simulink model "Aero_Workspace"  (R2021a)
settings: Solver=ode1be  StartTime=0.0  StopTime=inf  FixedStep=0.001  RelTol=1e-3  EnableMultiTasking=on
PreLoadFcn:
  | Aero_Workspace_Setup
model workspace (MAT data in the model file):
  Dg = 0.0071
  Dt = 0.158
  Jp = 0.022
  Mb = 1.3
  g = 9.81
values from neighbouring files (symbols this model uses):
  Kpp = 0.6*0.0154    (= 0.00924)    [Aero_Workspace_Parameters.m]
  Kpy = 2*0.00329    (= 0.00658)    [Aero_Workspace_Parameters.m]
  Kyp = -2.5*0.00167    (= -0.004175)    [Aero_Workspace_Parameters.m]
  Kyy = 0.0129    [Aero_Workspace_Parameters.m]
  Pitch_deg_range = 62    [Aero_Workspace_Setup.m]
undefined symbols (not defined in the file or in its folder): _AICAD8418WBRMZ_Default_sldprt, _AICBCR421UW67_Default_sldprt, _C0402100n25V_Default_sldprt, _C040210n25V_Default_sldprt, _C040212p50VC0G_Default_sldprt, _C06031u35V_Default_sldprt, _C06032u216V_Default_sldprt, _C100U50VEEEFC1H101P_Default_sldprt, _C12064u750V_01_sldprt, _C121010U50V_Default_sldprt, _COMMCYUSB2014BZXC_Default_sldprt, _COMMON_01_sldprt, _COMMON_Default_sldprt, _CONNFUSBBSMT_01_sldprt, _CONNMDF3A12P2DSA_Default_sldprt, _CONNMDF3A4P2DSA_Default_sldprt, _CONNMDF3A6P2DS_Default_sldprt, _CONNMDF3A9P2DS_Default_sldprt, _CONNMODULAR8P8CTOP_Default_sldprt, _CP6100U50VC0G_Default_sldprt, _CPLD5M80ZE64C5_Default_sldprt, _DB560C13F_01_sldprt, _Default_sldprt, _DSMBJ5361BTP_Default_sldprt, _EEPROMAT24CM01_Default_sldprt, _FBBLM21PG221SN1D_01_sldprt, _FBMPZ2012S601A_01_sldprt, _LED3mmRedGreenRA_Default_sldprt, _LEDLTRBGFSFRedGreenBlue_Default_sldprt, _LOGICNCP361SNT1G_Default_sldprt, _LOGICNOTSN74LVC3G14DCU_Default_sldprt, _OPL6206QTR_Default_sldprt, _OSC40000MHZ_Default_sldprt, _R0402100K_Default_sldprt, _R040210K0_Default_sldprt, _R04021K00_Default_sldprt, _R0402200R_Default_sldprt, _R040222R0_Default_sldprt, _R04026K04_Default_sldprt, _R0402DNP_Default_sldprt, _RA40R0_Default_sldprt, _RA41K005, _TP16258543_01_sldprt, _TVSUNI28V_Default_sldprt, _TVSUNI53V_Default_sldprt, _VREGAP733333SAG7_Default_sldprt, _VREGLTM8022EVPBF_Default_sldprt, _VREGPAM3112DAB120_Default_sldprt, _VREGTPS79318DBVR_01_sldprt, _XTAL192MHZNX2520SA_Default_sldprt, BGA121, CAP, CEEEFC1H101P, CONNFUSBBSMT, CONNMDF3A12P2DSA, CONNMDF3A4P2DSA, CONNMDF3A6P2DS, CONNMDF3A9P2DS, CONNModular8P8C, DDO214AA ... (+30)
libraries: sm_lib x1565, fl_lib x43, nesl_utility x22, quarc_library x12, simulink x2, ee_lib x2
(part 1 of 23)
settings Model: SimulationMode=external  ExtModeTrigDuration=10000  OrderedModelArguments=off  Creator=mbohra  LastModifiedBy=Derek
settings SolverCC: AlgebraicLoopSolver=TrustRegion  PositivePriorityOrder=on
settings DataIOCC: ReturnWorkspaceOutputs=off
settings DebuggingCC: SFMachineParentedDataDiag=warning  ArithmeticOperatorsInVariantConditions=warning
settings SFSimCC: SimUseLocalCustomCode=off  CustomCodeUndefinedFunction=UseInterfaceOnly
settings RTWCC: Description=QUARC Win64 Target Using Toolchain  SystemTargetFile=quarc_win64.tlc  TemplateMakefile=quarc_default_tmf  RTWUseLocalCustomCode=off  Toolchain=QUARC win64 | nmake (64-bit Windows)  BuildConfiguration=Faster Runs
settings CodeAppCC: StateflowObjectComments=on
settings STFCustomTargetCC: TargetLangStandard=C99 (ISO)  ConcurrentExecutionCompliant=on  SystemTargetFile=quarc_win64.tlc
settings GRTTargetCC: ParMdlRefBuildCompliant=off  CompOptLevelCompliant=off  CombineOutputUpdateFcns=off  MatFileLogging=off  CPPClassGenCompliant=off  GRTInterface=on  ExtMode=on  ExtModeMexFile=quarc_comm
settings ConfigComp: CovMetricSettings=dswe
settings ExplorerConfigSet: SimMechanicsOpenEditorOnUpdate=off

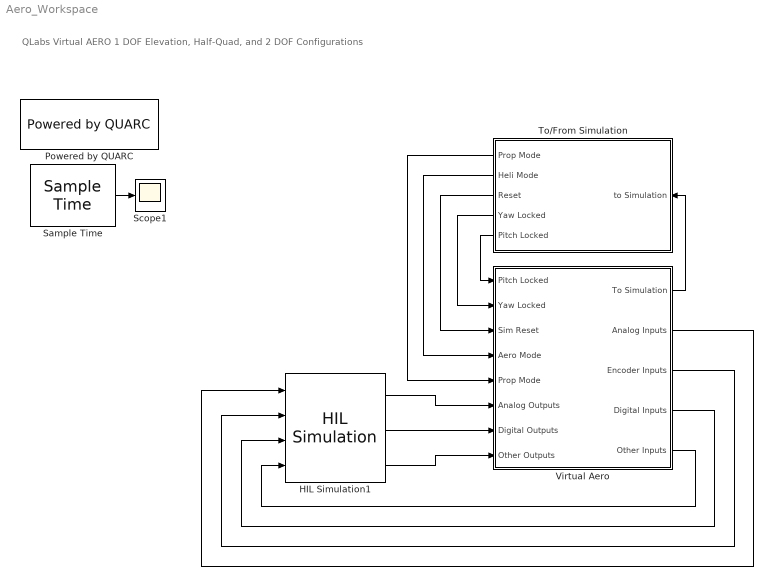
== system Aero_Workspace ==
  note: QLabs Virtual AERO
      | 1 DOF Elevation, Half-Quad, and 2 DOF Configurations
  HIL Simulation1 : quarc_library/Data Acquisition/Generic/Configuration/HIL Simulation  uri=tcpip://localhost:18930  board_type=quanser_aero_usb  board_id=0  sample_time=qc_get_step_size  active=on  num_clocks=1  num_interrupts=0  num_analog_inputs=2  num_analog_outputs=2  initial_analog=[]  num_digital_io=0  num_digital_inputs=3  num_digital_outputs=2  initial_digital=[]  num_encoder_inputs=4  num_pwm_outputs=0  initial_pwm=[]  other_inputs=[3000:3002 4000:4002 14000:14003]  other_outputs=[11000:11002]  initial_other=[]  integer_properties=[]  double_properties=[]  string_properties=[]
      settings: SourceProductName=QUARC Targets
  Powered by QUARC : quarc_library/Logos/Powered by QUARC
  Sample Time : quarc_library/Sources/Time/Sample Time  Priority=-99  sample_time=qc_get_step_size
  Scope1 : Scope
  To/From Simulation : Subsystem
  Virtual Aero : Subsystem
  wires:
  Virtual Aero/5(Other Inputs) -> HIL Simulation1/4
  Sample Time/1 -> Scope1/1
  Virtual Aero/2(Analog Inputs) -> HIL Simulation1/1
  Virtual Aero/3(Encoder Inputs) -> HIL Simulation1/2
  HIL Simulation1/1 -> Virtual Aero/6(Analog Outputs)
  HIL Simulation1/2 -> Virtual Aero/7(Digital Outputs)
  HIL Simulation1/3 -> Virtual Aero/8(Other Outputs)
  Virtual Aero/1(To Simulation) -> To/From Simulation/1(to Simulation)
  To/From Simulation/5(Pitch Locked) -> Virtual Aero/1(Pitch Locked)
  To/From Simulation/4(Yaw Locked) -> Virtual Aero/2(Yaw Locked)
  To/From Simulation/3(Reset) -> Virtual Aero/3(Sim Reset)
  To/From Simulation/2(Heli Mode) -> Virtual Aero/4(Aero Mode)
  To/From Simulation/1(Prop Mode) -> Virtual Aero/5(Prop Mode)
  Virtual Aero/4(Digital Inputs) -> HIL Simulation1/3

== system Aero_Workspace/To//From Simulation ==
  note: Yaw
      | Pitch
      | Motor 0 Speed
      | Motor 1 Speed
      | Base Color
  to Simulation : Inport
  "Connection State " : Scope  NumInputPorts=2
  Delay : Delay  DelayLength=1
  Delay1 : Delay  DelayLength=1
  Demux : Demux  Outputs=[1 1 1 1 3]
  Device Num : Constant  Value=0
  MATLAB Function : MATLAB Function  TreatAsAtomicUnit=on
  MATLAB Function1 : MATLAB Function  TreatAsAtomicUnit=on
  Memory : Memory
  "Reset Scope " : Scope
  SBS Error : Display
  Stream Server : quarc_library/Communications/Basic/Stream Server  uri_source=Specify via dialog (do not evaluate)  uri=tcpip://remotehost:18001?nagle='off'  apply_uri_to_all_configs=on  send_buffer_size=65537  receive_buffer_size=65537  byte_order=little endian (Intel - LSB first)  optimization=Minimum latency  send_options=Send all data  receive_options=Receive all data  default_value=[0]  sample_time=qc_get_step_size  active=on  implementation=Use blocking I/O in a separate thread  send_fifo_size=3  receive_fifo_size=3  send_priority=0  receive_priority=0  send_dimensions=on  receive_dimensions=on  max_dimensions=65537  data_type=uint8  type_expr=BusObject
      settings: AttributesFormatString="\"tcpip://remotehost:18001?nagle='off'\""
  Terminator1 : Terminator
  Prop Mode : Outport  OutDataTypeStr=double  VectorParamsAs1DForOutWhenUnconnected=off
  Heli Mode : Outport  Port=2  OutDataTypeStr=double  VectorParamsAs1DForOutWhenUnconnected=off
  Reset : Outport  Port=3  VectorParamsAs1DForOutWhenUnconnected=off
  Yaw Locked : Outport  Port=4  OutDataTypeStr=double  VectorParamsAs1DForOutWhenUnconnected=off
  Pitch Locked : Outport  Port=5  OutDataTypeStr=double  VectorParamsAs1DForOutWhenUnconnected=off
  wires:
  Stream Server/3 -> Terminator1/1
  MATLAB Function1/5(PropMode) -> Prop Mode/1
  Delay1/1 -> MATLAB Function/2(SendStateUpdate)
  MATLAB Function1/4(HeliMode) -> Heli Mode/1
  MATLAB Function1/6(Reset) -> Memory/1
  Memory/1 -> "Reset Scope "/1, Reset/1  "other returns"
  MATLAB Function/2(Enable) -> Stream Server/2
  Delay/1 -> MATLAB Function/1(ServerState)
  MATLAB Function/1(Packet) -> Stream Server/1
  MATLAB Function1/3(PitchLocked) -> Pitch Locked/1
  Stream Server/5 -> "Connection State "/2, MATLAB Function1/2(New)
  Stream Server/4 -> MATLAB Function1/1(Receive)
  MATLAB Function1/1(RequestServerUpdate) -> Delay1/1
  Stream Server/2 -> SBS Error/1
  MATLAB Function1/2(YawLocked) -> Yaw Locked/1
  Stream Server/1 -> Delay/1, "Connection State "/1
  Demux/5 -> MATLAB Function/8(BaseColor_v3)
  to Simulation/1 -> Demux/1
  Demux/1 -> MATLAB Function/4(Yaw)
  Demux/2 -> MATLAB Function/5(Pitch)
  Demux/3 -> MATLAB Function/6(Motor0Speed)
  Demux/4 -> MATLAB Function/7(Motor1Speed)
  Device Num/1 -> MATLAB Function/3(DeviceNumber)

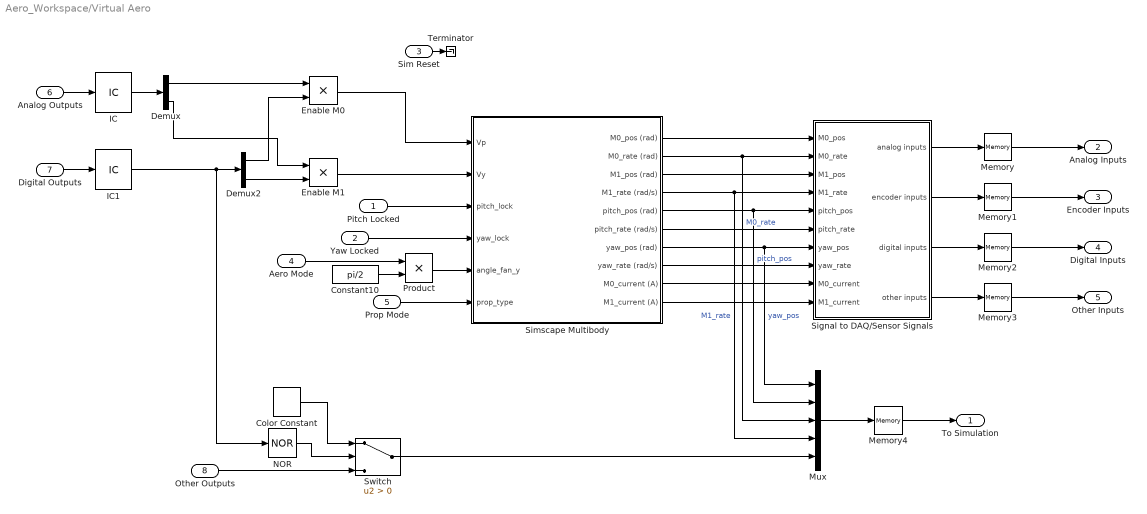
== system Aero_Workspace/Virtual Aero ==
  Pitch Locked : Inport
  Yaw Locked : Inport  Port=2
  Sim Reset : Inport  Port=3
  Aero Mode : Inport  Port=4
  Prop Mode : Inport  Port=5
  Analog Outputs : Inport  Port=6
  Digital Outputs : Inport  Port=7
  Other Outputs : Inport  Port=8
  Color Constant : quarc_library/Sources/Signals/Color Constant  color=[1 0 0]
      settings: SourceProductName=QUARC Targets
  Constant10 : Constant  Value=pi/2
  Demux : Demux  Outputs=2
  Demux2 : Demux  Outputs=2
  Enable M0 : Product
  Enable M1 : Product
  IC : InitialCondition  Value=0
  IC1 : InitialCondition  Value=0
  Memory{,1..4} (5 alike) : quarc_library/Discrete/Memory  initial_condition=0  sample_time=-1
      settings: SourceProductName=QUARC Targets
  Mux : Mux  Inputs=5
  NOR : Logic  Operator=NOR  Inputs=1  IconShape=distinctive  AllPortsSameDT=off  OutDataTypeStr=boolean
  Product : Product
  Signal to DAQ/Sensor Signals : Subsystem
  Simscape Multibody : Subsystem  VariantControl=Plant_Simscape
  Switch : Switch  Criteria=u2 > Threshold
  Terminator : Terminator
  To Simulation : Outport  VectorParamsAs1DForOutWhenUnconnected=off
  Analog Inputs : Outport  Port=2  VectorParamsAs1DForOutWhenUnconnected=off
  Encoder Inputs : Outport  Port=3  VectorParamsAs1DForOutWhenUnconnected=off
  Digital Inputs : Outport  Port=4
  Other Inputs : Outport  Port=5  VectorParamsAs1DForOutWhenUnconnected=off
  wires:
  Demux/1 -> Enable M0/1
  Demux2/1 -> Enable M0/2
  Demux/2 -> Enable M1/1
  Demux2/2 -> Enable M1/2
  Pitch Locked/1 -> Simscape Multibody/3(pitch_lock)
  Aero Mode/1 -> Product/1
  Constant10/1 -> Product/2
  Other Outputs/1 -> Switch/3
  Color Constant/1 -> Switch/1
  Switch/1 -> Mux/5
  Simscape Multibody/5(pitch_pos (rad)) -> Signal to DAQ/Sensor Signals/5(pitch_pos), Mux/2  "pitch_pos"
  Simscape Multibody/7(yaw_pos (rad)) -> Mux/1, Signal to DAQ/Sensor Signals/7(yaw_pos)  "yaw_pos"
  Simscape Multibody/2(M0_rate (rad)) -> Mux/3, Signal to DAQ/Sensor Signals/2(M0_rate)  "M0_rate"
  Simscape Multibody/4(M1_rate (rad/s)) -> Mux/4, Signal to DAQ/Sensor Signals/4(M1_rate)  "M1_rate"
  NOR/1 -> Switch/2
  Yaw Locked/1 -> Simscape Multibody/4(yaw_lock)
  Product/1 -> Simscape Multibody/5(angle_fan_y)
  Simscape Multibody/1(M0_pos (rad)) -> Signal to DAQ/Sensor Signals/1(M0_pos)
  Simscape Multibody/3(M1_pos (rad)) -> Signal to DAQ/Sensor Signals/3(M1_pos)
  Simscape Multibody/6(pitch_rate (rad/s)) -> Signal to DAQ/Sensor Signals/6(pitch_rate)
  Simscape Multibody/8(yaw_rate (rad/s)) -> Signal to DAQ/Sensor Signals/8(yaw_rate)
  Simscape Multibody/9(M0_current (A)) -> Signal to DAQ/Sensor Signals/9(M0_current)
  Simscape Multibody/10(M1_current (A)) -> Signal to DAQ/Sensor Signals/10(M1_current)
  Sim Reset/1 -> Terminator/1
  Signal to DAQ/Sensor Signals/1(analog inputs) -> Memory/1
  Memory/1 -> Analog Inputs/1
  Signal to DAQ/Sensor Signals/2(encoder inputs) -> Memory1/1
  Memory1/1 -> Encoder Inputs/1
  Signal to DAQ/Sensor Signals/3(digital inputs) -> Memory2/1
  Memory2/1 -> Digital Inputs/1
  Signal to DAQ/Sensor Signals/4(other inputs) -> Memory3/1
  Memory3/1 -> Other Inputs/1
  Mux/1 -> Memory4/1
  Memory4/1 -> To Simulation/1
  Digital Outputs/1 -> IC1/1
  Analog Outputs/1 -> IC/1
  Enable M1/1 -> Simscape Multibody/2(Vy)
  Enable M0/1 -> Simscape Multibody/1(Vp)
  Prop Mode/1 -> Simscape Multibody/6(prop_type)
  IC/1 -> Demux/1
  IC1/1 -> Demux2/1, NOR/1

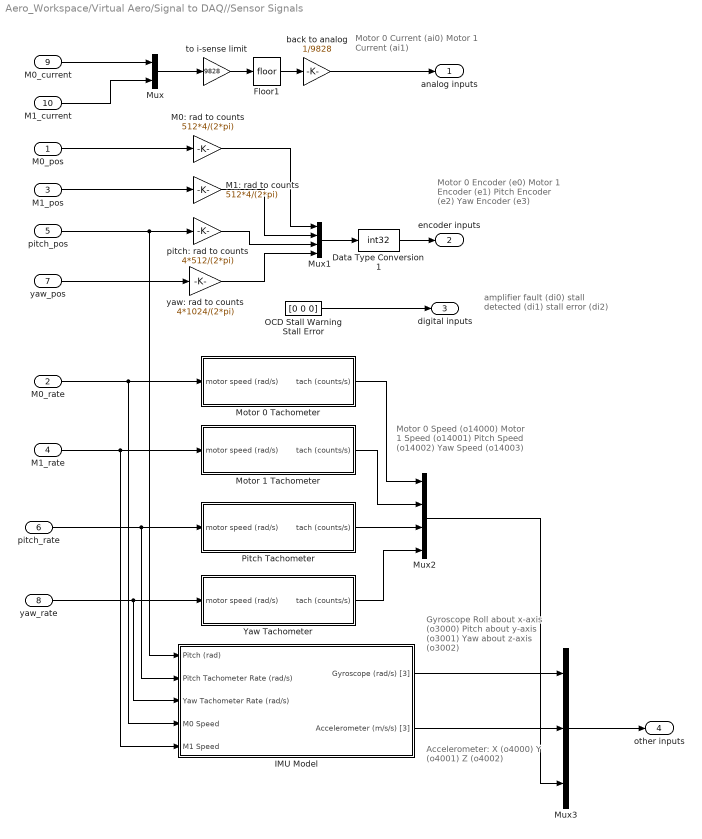
== system Aero_Workspace/Virtual Aero/Signal to DAQ//Sensor Signals ==
  note: Accelerometer:
      | X (o4000)
      | Y (o4001)
      | Z (o4002)
  note: Motor 0 Current (ai0)
      | Motor 1 Current (ai1)
  note: amplifier fault (di0)
      | stall detected (di1)
      | stall error (di2)
  note: Motor 0 Encoder (e0)
      | Motor 1 Encoder (e1)
      | Pitch Encoder (e2)
      | Yaw Encoder (e3)
  note: Motor 0 Speed (o14000)
      | Motor 1 Speed (o14001)
      | Pitch Speed (o14002)
      | Yaw Speed (o14003)
  note: Gyroscope
      | Roll about x-axis (o3000)
      | Pitch about y-axis (o3001)
      | Yaw about z-axis (o3002)
  M0_pos : Inport
  M0_rate : Inport  Port=2
  M1_pos : Inport  Port=3
  M1_rate : Inport  Port=4
  pitch_pos : Inport  Port=5
  pitch_rate : Inport  Port=6
  yaw_pos : Inport  Port=7
  yaw_rate : Inport  Port=8
  M0_current : Inport  Port=9
  M1_current : Inport  Port=10
  Data Type Conversion1 : DataTypeConversion  OutDataTypeStr=int32
  Floor1 : Rounding
  IMU Model : Subsystem
  M0: rad to counts : Gain  Gain=512*4/(2*pi)
  M1: rad to counts : Gain  Gain=512*4/(2*pi)
  Motor 0 Tachometer : Subsystem
  Motor 1 Tachometer : Subsystem
  Mux : Mux  Inputs=2
  Mux1 : Mux
  Mux2 : Mux
  Mux3 : Mux  Inputs=3
  OCD Stall Warning Stall Error : Constant  Value=[0 0 0]  OutDataTypeStr=boolean
  Pitch Tachometer : Subsystem
  Yaw Tachometer : Subsystem
  back to analog : Gain  Gain=1/9828
  pitch: rad to counts : Gain  Gain=4*512/(2*pi)
  to i-sense limit : Gain  Gain=9828
  yaw: rad to counts : Gain  Gain=4*1024/(2*pi)
  analog inputs : Outport
  encoder inputs : Outport  Port=2
  digital inputs : Outport  Port=3
  other inputs : Outport  Port=4
  wires:
  IMU Model/2(Accelerometer (m/s/s) [3]) -> Mux3/2
  IMU Model/1(Gyroscope (rad/s) [3]) -> Mux3/1
  Mux3/1 -> other inputs/1
  Mux2/1 -> Mux3/3
  Yaw Tachometer/1(tach (counts/s)) -> Mux2/4
  Pitch Tachometer/1(tach (counts/s)) -> Mux2/3
  Motor 1 Tachometer/1(tach (counts/s)) -> Mux2/2
  M1_rate/1 -> IMU Model/5(M1 Speed), Motor 1 Tachometer/1(motor speed (rad/s))
  pitch_rate/1 -> IMU Model/2(Pitch Tachometer Rate (rad/s)), Pitch Tachometer/1(motor speed (rad/s))
  yaw_rate/1 -> IMU Model/3(Yaw Tachometer Rate (rad/s)), Yaw Tachometer/1(motor speed (rad/s))
  M0_rate/1 -> IMU Model/4(M0 Speed), Motor 0 Tachometer/1(motor speed (rad/s))
  Data Type Conversion1/1 -> encoder inputs/1
  Mux1/1 -> Data Type Conversion1/1
  M0: rad to counts/1 -> Mux1/1
  M1: rad to counts/1 -> Mux1/2
  yaw: rad to counts/1 -> Mux1/4
  pitch: rad to counts/1 -> Mux1/3
  OCD Stall Warning Stall Error/1 -> digital inputs/1
  Floor1/1 -> back to analog/1
  to i-sense limit/1 -> Floor1/1
  Mux/1 -> to i-sense limit/1
  M0_pos/1 -> M0: rad to counts/1
  yaw_pos/1 -> yaw: rad to counts/1
  pitch_pos/1 -> IMU Model/1("Pitch (rad) "), pitch: rad to counts/1
  M1_pos/1 -> M1: rad to counts/1
  M0_current/1 -> Mux/1
  M1_current/1 -> Mux/2
  Motor 0 Tachometer/1(tach (counts/s)) -> Mux2/1
  back to analog/1 -> analog inputs/1

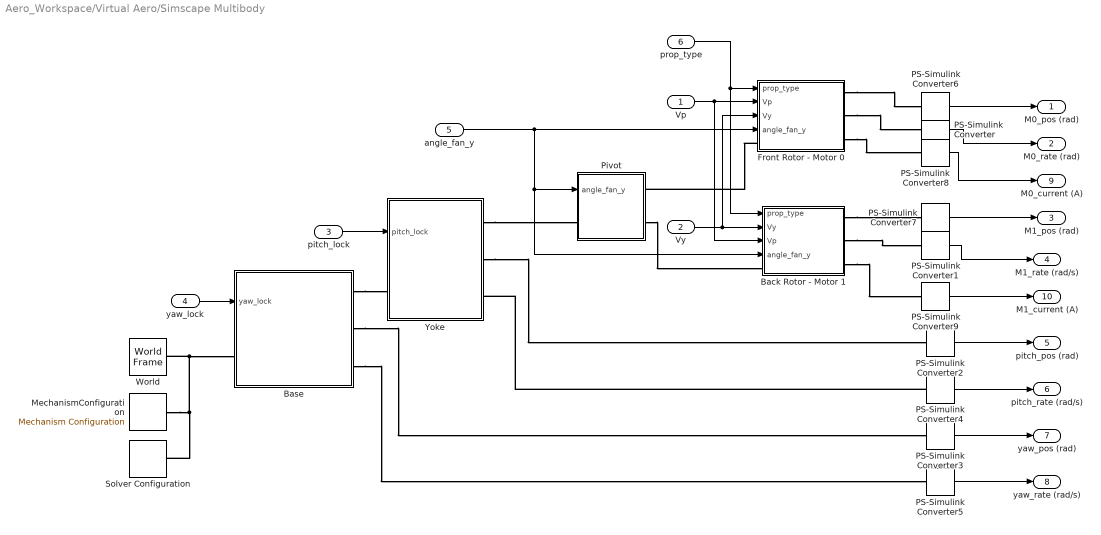
== system Aero_Workspace/Virtual Aero/Simscape Multibody ==
  Vp : Inport
  Vy : Inport  Port=2
  pitch_lock : Inport  Port=3
  yaw_lock : Inport  Port=4
  angle_fan_y : Inport  Port=5
  prop_type : Inport  Port=6
  Back Rotor - Motor 1 : Subsystem
  Base : Subsystem
      mask Display: image('Base.jpg')
  "Front Rotor - Motor 0  " : Subsystem
  MechanismConfiguration : sm_lib/Utilities/Mechanism Configuration  UniformGravity=Constant  GravityVector=[0 -9.81 0]  GravityVectorUnits=m/s^2  GravityUnits=m/s^2  LinearizationDelta=0.001  JointModeTransitionNonlinearIterations=2
  PS-Simulink Converter{,1,4..5} (4 alike) : nesl_utility/PS-Simulink Converter  PhysicalDomain=network_engine_domain  SubClassName=ps_output  LeftPortType=input  RightPortType=output  PseudoPeriodic=off  Frequencies=[]  Unit=rad/s  AffineConversion=off
      settings: SourceProductBaseCode=PW,SS
  PS-Simulink Converter{2..3,6..7} (4 alike) : nesl_utility/PS-Simulink Converter  PhysicalDomain=network_engine_domain  SubClassName=ps_output  LeftPortType=input  RightPortType=output  PseudoPeriodic=off  Frequencies=[]  Unit=rad  AffineConversion=off
      settings: SourceProductBaseCode=PW,SS
  PS-Simulink Converter8 : nesl_utility/PS-Simulink Converter  PhysicalDomain=network_engine_domain  SubClassName=ps_output  LeftPortType=input  RightPortType=output  PseudoPeriodic=off  Frequencies=[]  Unit=A  AffineConversion=off
      settings: SourceProductBaseCode=PW,SS
  PS-Simulink Converter9 : nesl_utility/PS-Simulink Converter  PhysicalDomain=network_engine_domain  SubClassName=ps_output  LeftPortType=input  RightPortType=output  PseudoPeriodic=off  Frequencies=[]  Unit=A  AffineConversion=off
      settings: SourceProductBaseCode=PW,SS
  Pivot : Subsystem
  Solver Configuration : nesl_utility/Solver Configuration  PhysicalDomain=network_engine_domain  SubClassName=solver  LeftPortType=input  RightPortType=generic  Tones=[]  Harmonics=[]  SimulateNoise=off  Profile=off  UseLocalSampling=off  EnableSwitchedLinearOptims=on  FrequencyDomain=off  UseCCode=off  RelTol=0.001  AbsTol=1e-06  MinStep=1e-09  ToWorkspace=off  RevertToSquareIcSolve=off  NumHomotopyIterations=100  PhasorMode=off  PhasorModeNumHarmonics=1  DoDC=off  ResidualTolerance=1e-09  UseLocalSolver=off  LocalSolverChoice=NE_BACKWARD_EULER_ADVANCER  LocalSolverSampleTime=1e-3  DoFixedCost=off  MaxNonlinIter=3  MaxModeIter=2  ComputeImpulses=off  ImpulseIterations=2  LinearAlgebra=Sparse  EquationFormulation=NE_TIME_EF  DelaysMemoryBudget=1024  AutomaticFiltering=on  FilteringTimeConstant=0.001  PartitionStorageMethod=AS_NEEDED  PartitionMemoryBudget=1024  PartitionMethod=FAST
      settings: SourceProductBaseCode=PW,SS
  World : sm_lib/Frames and Transforms/World Frame
  Yoke : Subsystem
  M0_pos (rad) : Outport
  M0_rate (rad) : Outport  Port=2
  M1_pos (rad) : Outport  Port=3
  M1_rate (rad/s) : Outport  Port=4
  pitch_pos (rad) : Outport  Port=5
  pitch_rate (rad/s) : Outport  Port=6
  yaw_pos (rad) : Outport  Port=7
  yaw_rate (rad/s) : Outport  Port=8
  M0_current (A) : Outport  Port=9
  M1_current (A) : Outport  Port=10
  wires:
  Vy/1 -> "Front Rotor - Motor 0  "/3(Vy), Back Rotor - Motor 1/2(Vy)
  Vp/1 -> Back Rotor - Motor 1/3(Vp), "Front Rotor - Motor 0  "/2(Vp)
  pitch_lock/1 -> Yoke/1(pitch_lock)
  yaw_lock/1 -> Base/1(yaw_lock)
  angle_fan_y/1 -> "Front Rotor - Motor 0  "/4(angle_fan_y), Pivot/1(angle_fan_y), Back Rotor - Motor 1/4(angle_fan_y)
  PS-Simulink Converter6/1 -> M0_pos (rad)/1
  PS-Simulink Converter7/1 -> M1_pos (rad)/1
  PS-Simulink Converter1/1 -> M1_rate (rad/s)/1
  PS-Simulink Converter2/1 -> pitch_pos (rad)/1
  PS-Simulink Converter4/1 -> pitch_rate (rad/s)/1
  PS-Simulink Converter3/1 -> yaw_pos (rad)/1
  PS-Simulink Converter5/1 -> yaw_rate (rad/s)/1
  PS-Simulink Converter8/1 -> M0_current (A)/1
  PS-Simulink Converter9/1 -> M1_current (A)/1
  PS-Simulink Converter/1 -> M0_rate (rad)/1
  prop_type/1 -> Back Rotor - Motor 1/1(prop_type), "Front Rotor - Motor 0  "/1(prop_type)
  connections:
  MechanismConfiguration/RConn1 -- Base/LConn1 -- World/RConn1 -- Solver Configuration/RConn1
  Yoke/RConn1 -- Pivot/LConn1
  Base/RConn1 -- Yoke/LConn1
  "Front Rotor - Motor 0  "/LConn1 -- Pivot/RConn1
  Pivot/RConn2 -- Back Rotor - Motor 1/LConn1
  "Front Rotor - Motor 0  "/RConn1 -- PS-Simulink Converter6/LConn1
  Back Rotor - Motor 1/RConn1 -- PS-Simulink Converter7/LConn1
  Yoke/RConn2 -- PS-Simulink Converter2/LConn1
  Base/RConn2 -- PS-Simulink Converter3/LConn1
  "Front Rotor - Motor 0  "/RConn2 -- PS-Simulink Converter/LConn1
  Back Rotor - Motor 1/RConn2 -- PS-Simulink Converter1/LConn1
  PS-Simulink Converter4/LConn1 -- Yoke/RConn3
  Base/RConn3 -- PS-Simulink Converter5/LConn1
  "Front Rotor - Motor 0  "/RConn3 -- PS-Simulink Converter8/LConn1
  Back Rotor - Motor 1/RConn3 -- PS-Simulink Converter9/LConn1

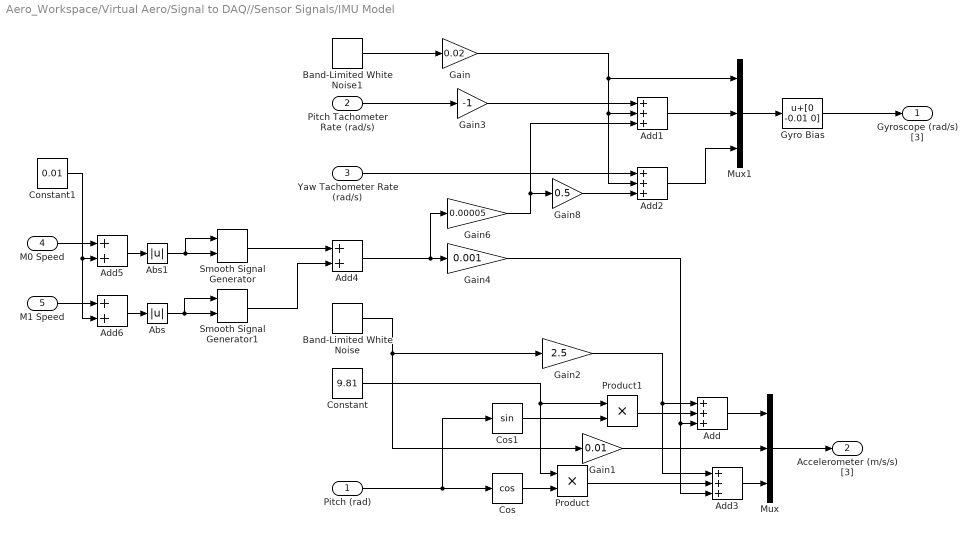
== system Aero_Workspace/Virtual Aero/Signal to DAQ//Sensor Signals/IMU Model ==
  "Pitch (rad) " : Inport
  Pitch Tachometer Rate (rad/s) : Inport  Port=2
  Yaw Tachometer Rate (rad/s) : Inport  Port=3
  M0 Speed : Inport  Port=4
  M1 Speed : Inport  Port=5
  Abs : Abs
  Abs1 : Abs
  Add{,1..3} (4 alike) : Sum  Inputs=+++
  Add4 : Sum
  Add5 : Sum
  Add6 : Sum
  Band-Limited White Noise : simulink/Sources/Band-Limited White Noise  Cov=[0.00001]  Ts=qc_get_step_size  seed=randi(10000, 1)
  Band-Limited White Noise1 : simulink/Sources/Band-Limited White Noise  Cov=[0.00001]  Ts=qc_get_step_size  seed=randi(10000, 1)
  Constant : Constant  Value=9.81
  Constant1 : Constant  Value=0.01
  Cos : Trigonometry  Operator=cos
  Cos1 : Trigonometry
  Gain : Gain  Gain=0.02
  Gain1 : Gain  Gain=0.01
  Gain2 : Gain  Gain=2.5
  Gain3 : Gain  Gain=-1
  Gain4 : Gain  Gain=0.001
  Gain6 : Gain  Gain=0.00005
  Gain8 : Gain  Gain=0.5
  Gyro Bias : Bias  Bias=[0 -0.01 0]
  Mux : Mux  Inputs=3
  Mux1 : Mux  Inputs=3
  Product : Product
  Product1 : Product
  Smooth Signal Generator : quarc_library/Sources/Signals/Smooth Signal Generator  signal_type=Sine  source=External (input ports)  amplitude=1  frequency=1  initial_phase=0  sample_time=qc_get_step_size  output_cos=off
      settings: SourceProductName=QUARC Targets
  Smooth Signal Generator1 : quarc_library/Sources/Signals/Smooth Signal Generator  signal_type=Sine  source=External (input ports)  amplitude=1  frequency=1  initial_phase=0  sample_time=qc_get_step_size  output_cos=off
      settings: SourceProductName=QUARC Targets
  Gyroscope (rad/s) [3] : Outport  VectorParamsAs1DForOutWhenUnconnected=off
  Accelerometer (m/s/s) [3] : Outport  Port=2  VectorParamsAs1DForOutWhenUnconnected=off
  wires:
  Gain2/1 -> Add/1, Add3/1
  Gain/1 -> Add2/2, Add1/2, Mux1/1
  Mux/1 -> Accelerometer (m/s/s) [3]/1
  Add2/1 -> Mux1/3
  Yaw Tachometer Rate (rad/s)/1 -> Add2/1
  Cos/1 -> Product/2
  Cos1/1 -> Product1/2
  Constant/1 -> Product/1, Product1/1
  "Pitch (rad) "/1 -> Cos/1, Cos1/1
  Band-Limited White Noise/1 -> Gain2/1, Gain1/1
  Band-Limited White Noise1/1 -> Gain/1
  Pitch Tachometer Rate (rad/s)/1 -> Gain3/1
  Mux1/1 -> Gyro Bias/1
  Gain1/1 -> Mux/2
  Product1/1 -> Add/2
  Add/1 -> Mux/1
  Product/1 -> Add3/2
  Add3/1 -> Mux/3
  Gain3/1 -> Add1/1
  Smooth Signal Generator1/1 -> Add4/2
  Smooth Signal Generator/1 -> Add4/1
  Add4/1 -> Gain6/1, Gain4/1
  M0 Speed/1 -> Add5/1
  Constant1/1 -> Add6/2, Add5/2
  M1 Speed/1 -> Add6/1
  Gain8/1 -> Add2/3
  Gain6/1 -> Add1/3, Gain8/1
  Gain4/1 -> Add/3, Add3/3
  Add5/1 -> Abs1/1
  Add6/1 -> Abs/1
  Abs/1 -> Smooth Signal Generator1/1, Smooth Signal Generator1/2
  Abs1/1 -> Smooth Signal Generator/1, Smooth Signal Generator/2
  Add1/1 -> Mux1/2
  Gyro Bias/1 -> Gyroscope (rad/s) [3]/1

== system Aero_Workspace/Virtual Aero/Signal to DAQ//Sensor Signals/Motor 0 Tachometer ==
  note: the lowest reading on the tach
      | is +/-20 counts per second.
  motor speed (rad/s) : Inport
  Constant : Constant  Value=20
  Floor2 : Rounding
  M0: rad/s to counts/s : Gain  Gain=512*4/(2*pi)
  MATLAB Function : MATLAB Function  TreatAsAtomicUnit=on
  back to rads : Gain  Gain=1/2^24
  to datatype limit : Gain  Gain=2^24
  tach (counts/s) : Outport
  wires:
  M0: rad/s to counts/s/1 -> MATLAB Function/1(u)
  back to rads/1 -> M0: rad/s to counts/s/1
  Constant/1 -> MATLAB Function/2(t)
  to datatype limit/1 -> Floor2/1
  motor speed (rad/s)/1 -> to datatype limit/1
  MATLAB Function/1(y) -> tach (counts/s)/1
  Floor2/1 -> back to rads/1

== system Aero_Workspace/Virtual Aero/Signal to DAQ//Sensor Signals/Motor 1 Tachometer ==
  note: the lowest reading on the tach
      | is +/-20 counts per second.
  motor speed (rad/s) : Inport
  Constant : Constant  Value=20
  Floor2 : Rounding
  M1: rad/s to counts/s : Gain  Gain=512*4/(2*pi)
  MATLAB Function : MATLAB Function  TreatAsAtomicUnit=on
  back to rads : Gain  Gain=1/2^24
  to datatype limit : Gain  Gain=2^24
  tach (counts/s) : Outport
  wires:
  Floor2/1 -> back to rads/1
  MATLAB Function/1(y) -> tach (counts/s)/1
  motor speed (rad/s)/1 -> to datatype limit/1
  to datatype limit/1 -> Floor2/1
  Constant/1 -> MATLAB Function/2(t)
  back to rads/1 -> M1: rad/s to counts/s/1
  M1: rad/s to counts/s/1 -> MATLAB Function/1(u)

== system Aero_Workspace/Virtual Aero/Signal to DAQ//Sensor Signals/Pitch Tachometer ==
  note: the lowest reading on the tach
      | is +/-20 counts per second.
  motor speed (rad/s) : Inport
  Constant : Constant  Value=20
  Floor2 : Rounding
  MATLAB Function : MATLAB Function  TreatAsAtomicUnit=on
  back to rads : Gain  Gain=1/2^24
  pitch: rad/s to counts/s : Gain  Gain=4*512/(2*pi)
  to datatype limit : Gain  Gain=2^24
  tach (counts/s) : Outport
  wires:
  Constant/1 -> MATLAB Function/2(t)
  MATLAB Function/1(y) -> tach (counts/s)/1
  pitch: rad/s to counts/s/1 -> MATLAB Function/1(u)
  back to rads/1 -> pitch: rad/s to counts/s/1
  to datatype limit/1 -> Floor2/1
  motor speed (rad/s)/1 -> to datatype limit/1
  Floor2/1 -> back to rads/1

== system Aero_Workspace/Virtual Aero/Signal to DAQ//Sensor Signals/Yaw Tachometer ==
  note: the lowest reading on the tach
      | is +/-20 counts per second.
  motor speed (rad/s) : Inport
  Constant : Constant  Value=20
  Floor2 : Rounding
  MATLAB Function : MATLAB Function  TreatAsAtomicUnit=on
  back to rads : Gain  Gain=1/2^24
  to datatype limit : Gain  Gain=2^24
  yaw: rad/s to counts/s : Gain  Gain=4*1024/(2*pi)
  tach (counts/s) : Outport
  wires:
  Floor2/1 -> back to rads/1
  MATLAB Function/1(y) -> tach (counts/s)/1
  motor speed (rad/s)/1 -> to datatype limit/1
  to datatype limit/1 -> Floor2/1
  Constant/1 -> MATLAB Function/2(t)
  back to rads/1 -> yaw: rad/s to counts/s/1
  yaw: rad/s to counts/s/1 -> MATLAB Function/1(u)

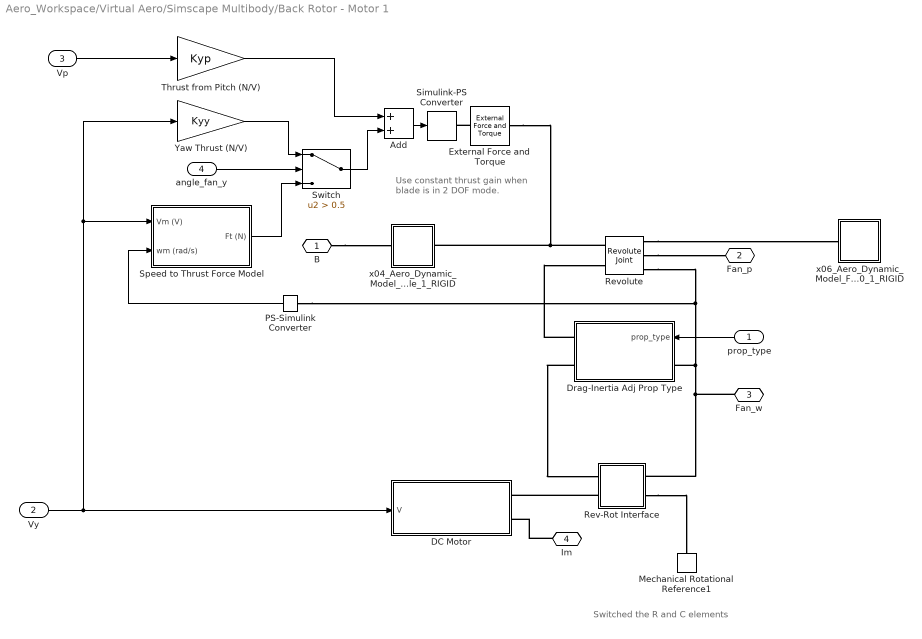
== system Aero_Workspace/Virtual Aero/Simscape Multibody/Back Rotor - Motor 1 ==
  note: Use constant thrust gain when
      | blade is in 2 DOF mode.
  note: Switched the R and C elements
  prop_type : Inport
  Vy : Inport  Port=2
  Vp : Inport  Port=3
  angle_fan_y : Inport  Port=4
  Add : Sum
  DC Motor : Subsystem
  Drag-Inertia Adj Prop Type : Subsystem
  External Force and Torque : sm_lib/Forces and Torques/External Force and Torque  ForceResolutionFrame=AttachedFrame  EnableForceX=off  EnableForceY=off  EnableForceZ=on  EnableForce=off  TorqueResolutionFrame=AttachedFrame  EnableTorqueX=off  EnableTorqueY=off  EnableTorqueZ=off  EnableTorque=off
  Mechanical Rotational Reference1 : fl_lib/Mechanical/Rotational Elements/Mechanical Rotational Reference
  PS-Simulink Converter : nesl_utility/PS-Simulink Converter  PhysicalDomain=network_engine_domain  SubClassName=ps_output  LeftPortType=input  RightPortType=output  PseudoPeriodic=off  Frequencies=[]  Unit=inherit  AffineConversion=off
      settings: SourceProductBaseCode=PW,SS
  Rev-Rot Interface : Subsystem
  Revolute : sm_lib/Joints/Revolute Joint  JointMode=Normal  SenseConstraintForce=off  SenseConstraintForceX=off  SenseConstraintForceY=off  SenseConstraintForceZ=off  SenseConstraintTorque=off  SenseConstraintTorqueX=off  SenseConstraintTorqueY=off  SenseConstraintTorqueZ=off  SenseTotalForce=off  SenseTotalForceX=off  SenseTotalForceY=off  SenseTotalForceZ=off  SenseTotalTorque=off  SenseTotalTorqueX=off  SenseTotalTorqueY=off  SenseTotalTorqueZ=off  CompositeWrenchDir=FollowerOnBase  CompositeWrenchFrame=BaseFrame  EquilibriumPosition=0  EquilibriumPositionUnits=rad  SpringStiffness=0  SpringStiffnessUnits=m*N/rad  DampingCoefficient=D_motor  DampingCoefficientUnits=m*s*N/rad  TorqueActuationMode=InputTorque  MotionActuationMode=ComputedMotion  SensePosition=on  SenseVelocity=on  SenseAcceleration=off  SenseTorqueForce=off  SenseLowerLimitTorqueForce=off  SenseUpperLimitTorqueForce=off  LowerLimitSpecify=off  LowerLimitBound=-90  LowerLimitBoundUnits=deg  LowerLimitStiffness=1e4  LowerLimitStiffnessUnits=N*m/deg  LowerLimitDamping=10  LowerLimitDampingUnits=N*m/(deg/s)  LowerLimitTransitionRegionWidth=0.1  LowerLimitTransitionRegionWidthUnits=deg  UpperLimitSpecify=off  UpperLimitBound=90  UpperLimitBoundUnits=deg  UpperLimitStiffness=1e4  UpperLimitStiffnessUnits=N*m/deg  UpperLimitDamping=10  UpperLimitDampingUnits=N*m/(deg/s)  UpperLimitTransitionRegionWidth=0.1  UpperLimitTransitionRegionWidthUnits=deg  PositionTargetSpecify=on  PositionTargetPriority=Low  PositionTargetValue=smiData.RevoluteJoint(1).Rz.Pos  PositionTargetValueUnits=deg  VelocityTargetSpecify=off  VelocityTargetPriority=High  VelocityTargetValue=0  VelocityTargetValueUnits=deg/s
  Simulink-PS Converter : nesl_utility/Simulink-PS Converter  PhysicalDomain=network_engine_domain  SubClassName=ps_input  LeftPortType=input  RightPortType=output  PseudoPeriodic=off  Frequencies=[]  NoiseDistribution=none  NoiseParameters=[]  Unit=1  AffineConversion=off  FilteringAndDerivatives=zero  SimscapeFilterOrder=1  InputFilterTimeConstant=0.001  UdotUserProvided=1
      settings: SourceProductBaseCode=PW,SS
  Speed to Thrust Force Model : Subsystem
  Switch : Switch  Criteria=u2 > Threshold  Threshold=0.5
  Thrust from Pitch (N/V) : Gain  Gain=Kyp
  Yaw Thrust (N/V) : Gain  Gain=Kyy
  x04_Aero_Dynamic_Model_Fan_0_Module_1_RIGID : Subsystem
  x06_Aero_Dynamic_Model_Fan_0_1_RIGID : Subsystem
  B : PMIOPort  Side=Left
  Fan_p : PMIOPort  Port=2  Side=Right
  Fan_w : PMIOPort  Port=3  Side=Right
  Im : PMIOPort  Port=4  Side=Right
  wires:
  prop_type/1 -> Drag-Inertia Adj Prop Type/1(prop_type)
  Add/1 -> Simulink-PS Converter/1
  Thrust from Pitch (N/V)/1 -> Add/1
  Vp/1 -> Thrust from Pitch (N/V)/1
  Vy/1 -> Yaw Thrust (N/V)/1, Speed to Thrust Force Model/1(Vm (V)), DC Motor/1(V)
  PS-Simulink Converter/1 -> Speed to Thrust Force Model/2(wm (rad/s))
  angle_fan_y/1 -> Switch/2
  Speed to Thrust Force Model/1(Ft (N)) -> Switch/3
  Switch/1 -> Add/2
  Yaw Thrust (N/V)/1 -> Switch/1
  connections:
  Drag-Inertia Adj Prop Type/RConn1 -- Revolute/LConn2
  Revolute/RConn3 -- PS-Simulink Converter/LConn1 -- Drag-Inertia Adj Prop Type/LConn1 -- Fan_w/RConn1 -- Rev-Rot Interface/RConn1
  Drag-Inertia Adj Prop Type/RConn2 -- Rev-Rot Interface/LConn1
  Im/RConn1 -- DC Motor/RConn2
  Rev-Rot Interface/LConn2 -- DC Motor/RConn1
  Revolute/RConn2 -- Fan_p/RConn1
  External Force and Torque/LConn1 -- Simulink-PS Converter/RConn1
  Revolute/LConn1 -- External Force and Torque/RConn1 -- x04_Aero_Dynamic_Model_Fan_0_Module_1_RIGID/RConn1
  B/RConn1 -- x04_Aero_Dynamic_Model_Fan_0_Module_1_RIGID/LConn1
  Rev-Rot Interface/RConn2 -- Mechanical Rotational Reference1/LConn1
  Revolute/RConn1 -- x06_Aero_Dynamic_Model_Fan_0_1_RIGID/LConn1

== system Aero_Workspace/Virtual Aero/Simscape Multibody/Base ==
  yaw_lock : Inport
  Transform : sm_lib/Frames and Transforms/Rigid Transform  TranslationMethod=Cartesian  TranslationStandardOffset=0  TranslationLengthUnit=in  TranslationStandardAxis=+Z  TranslationCartesianOffset=smiData.RigidTransform(642).translation  TranslationROffset=0  TranslationROffsetUnits=m  TranslationZOffset=0  TranslationZOffsetUnits=m  TranslationThetaOffset=0  TranslationThetaOffsetUnits=deg  RotationMethod=ArbitraryAxis  RotationAngleUnits=rad  RotationStandardAxis=+Z  RotationAngle=smiData.RigidTransform(642).angle  RotationArbitraryAxis=smiData.RigidTransform(642).axis  FollAlignAxisA=+X  BaseAlignAxisA=+Y  FollAlignAxisB=+Y  BaseAlignAxisB=+Z  RotationSequenceAxes=FollowerAxes  RotationSequence=XYX  RotationSequenceAngles=[0 0 0]  RotationSequenceAnglesUnits=deg  RotationMatrix=[1 0 0; 0 1 0; 0 0 1]
  Yaw Axis Rotation : Subsystem  VariantControl=Yaw_Unlocked
  x01_Aero_Dynamic_Model_Base_1_RIGID : Subsystem
  B : PMIOPort  Side=Left
  F : PMIOPort  Port=2  Side=Right
  Yaw_p : PMIOPort  Port=3  Side=Right
  Yaw_w : PMIOPort  Port=4  Side=Right
  wires:
  yaw_lock/1 -> Yaw Axis Rotation/1(yaw_lock)
  connections:
  Yaw Axis Rotation/RConn3 -- Yaw_w/RConn1
  Yaw Axis Rotation/RConn2 -- Yaw_p/RConn1
  Yaw Axis Rotation/LConn1 -- x01_Aero_Dynamic_Model_Base_1_RIGID/RConn1
  Yaw Axis Rotation/RConn1 -- F/RConn1
  Transform/RConn1 -- x01_Aero_Dynamic_Model_Base_1_RIGID/LConn1
  B/RConn1 -- Transform/LConn1

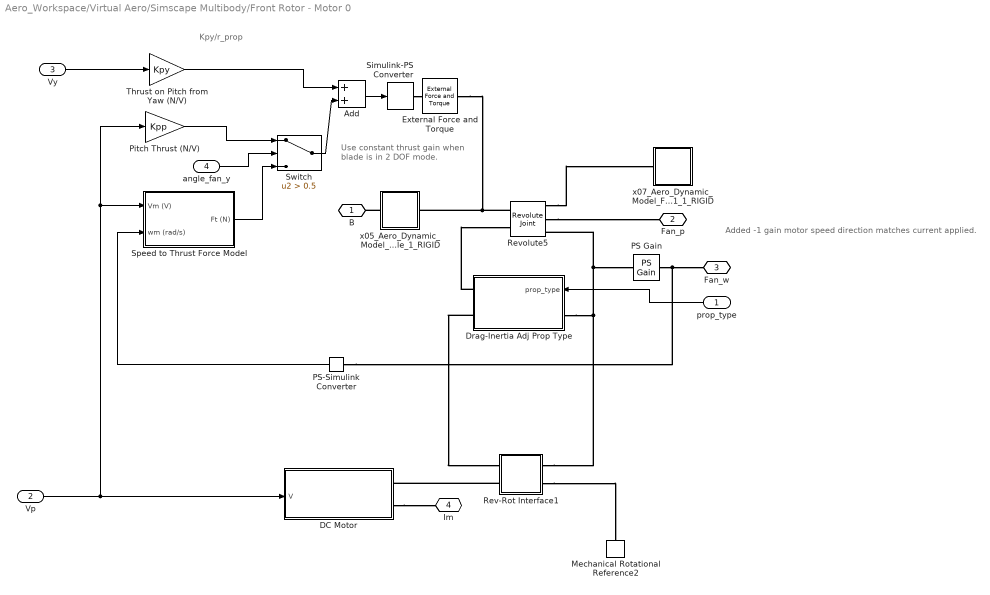
== system Aero_Workspace/Virtual Aero/Simscape Multibody/Front Rotor - Motor 0   ==
  note: Kpy/r_prop
  note: Added -1 gain motor speed direction matches current applied.
  note: Use constant thrust gain when
      | blade is in 2 DOF mode.
  prop_type : Inport
  Vp : Inport  Port=2
  Vy : Inport  Port=3
  angle_fan_y : Inport  Port=4
  Add : Sum  Inputs=2
  DC Motor : Subsystem
  Drag-Inertia Adj Prop Type : Subsystem
  External Force and Torque : sm_lib/Forces and Torques/External Force and Torque  ForceResolutionFrame=AttachedFrame  EnableForceX=off  EnableForceY=off  EnableForceZ=on  EnableForce=off  TorqueResolutionFrame=AttachedFrame  EnableTorqueX=off  EnableTorqueY=off  EnableTorqueZ=off  EnableTorque=off
  Mechanical Rotational Reference2 : fl_lib/Mechanical/Rotational Elements/Mechanical Rotational Reference
  PS Gain : fl_lib/Physical Signals/Functions/PS Gain  gain=-1
  PS-Simulink Converter : nesl_utility/PS-Simulink Converter  PhysicalDomain=network_engine_domain  SubClassName=ps_output  LeftPortType=input  RightPortType=output  PseudoPeriodic=off  Frequencies=[]  Unit=inherit  AffineConversion=off
      settings: SourceProductBaseCode=PW,SS
  Pitch Thrust (N/V) : Gain  Gain=Kpp
  Rev-Rot Interface1 : Subsystem
  Revolute5 : sm_lib/Joints/Revolute Joint  JointMode=Normal  SenseConstraintForce=off  SenseConstraintForceX=off  SenseConstraintForceY=off  SenseConstraintForceZ=off  SenseConstraintTorque=off  SenseConstraintTorqueX=off  SenseConstraintTorqueY=off  SenseConstraintTorqueZ=off  SenseTotalForce=off  SenseTotalForceX=off  SenseTotalForceY=off  SenseTotalForceZ=off  SenseTotalTorque=off  SenseTotalTorqueX=off  SenseTotalTorqueY=off  SenseTotalTorqueZ=off  CompositeWrenchDir=FollowerOnBase  CompositeWrenchFrame=BaseFrame  EquilibriumPosition=0  EquilibriumPositionUnits=rad  SpringStiffness=0  SpringStiffnessUnits=m*N/rad  DampingCoefficient=D_motor  DampingCoefficientUnits=N*m/(rad/s)  TorqueActuationMode=InputTorque  MotionActuationMode=ComputedMotion  SensePosition=on  SenseVelocity=on  SenseAcceleration=off  SenseTorqueForce=off  SenseLowerLimitTorqueForce=off  SenseUpperLimitTorqueForce=off  LowerLimitSpecify=off  LowerLimitBound=-90  LowerLimitBoundUnits=deg  LowerLimitStiffness=1e4  LowerLimitStiffnessUnits=N*m/deg  LowerLimitDamping=10  LowerLimitDampingUnits=N*m/(deg/s)  LowerLimitTransitionRegionWidth=0.1  LowerLimitTransitionRegionWidthUnits=deg  UpperLimitSpecify=off  UpperLimitBound=90  UpperLimitBoundUnits=deg  UpperLimitStiffness=1e4  UpperLimitStiffnessUnits=N*m/deg  UpperLimitDamping=10  UpperLimitDampingUnits=N*m/(deg/s)  UpperLimitTransitionRegionWidth=0.1  UpperLimitTransitionRegionWidthUnits=deg  PositionTargetSpecify=on  PositionTargetPriority=Low  PositionTargetValue=smiData.RevoluteJoint(6).Rz.Pos  PositionTargetValueUnits=deg  VelocityTargetSpecify=off  VelocityTargetPriority=High  VelocityTargetValue=0  VelocityTargetValueUnits=deg/s
  Simulink-PS Converter : nesl_utility/Simulink-PS Converter  PhysicalDomain=network_engine_domain  SubClassName=ps_input  LeftPortType=input  RightPortType=output  PseudoPeriodic=off  Frequencies=[]  NoiseDistribution=none  NoiseParameters=[]  Unit=1  AffineConversion=off  FilteringAndDerivatives=zero  SimscapeFilterOrder=1  InputFilterTimeConstant=0.001  UdotUserProvided=1
      settings: SourceProductBaseCode=PW,SS
  Speed to Thrust Force Model : Subsystem
  Switch : Switch  Criteria=u2 > Threshold  Threshold=0.5
  Thrust on Pitch from Yaw (N/V) : Gain  Gain=Kpy
  x05_Aero_Dynamic_Model_Fan_1_Module_1_RIGID : Subsystem
  x07_Aero_Dynamic_Model_Fan_1_1_RIGID : Subsystem
  B : PMIOPort  Side=Left
  Fan_p : PMIOPort  Port=2  Side=Right
  Fan_w : PMIOPort  Port=3  Side=Right
  Im : PMIOPort  Port=4  Side=Right
  wires:
  prop_type/1 -> Drag-Inertia Adj Prop Type/1(prop_type)
  Add/1 -> Simulink-PS Converter/1
  Thrust on Pitch from Yaw (N/V)/1 -> Add/1
  Vp/1 -> DC Motor/1(V), Pitch Thrust (N/V)/1, Speed to Thrust Force Model/1(Vm (V))
  Vy/1 -> Thrust on Pitch from Yaw (N/V)/1
  PS-Simulink Converter/1 -> Speed to Thrust Force Model/2(wm (rad/s))
  angle_fan_y/1 -> Switch/2
  Speed to Thrust Force Model/1(Ft (N)) -> Switch/3
  Switch/1 -> Add/2
  Pitch Thrust (N/V)/1 -> Switch/1
  connections:
  Drag-Inertia Adj Prop Type/RConn1 -- Revolute5/LConn2
  Revolute5/RConn1 -- x07_Aero_Dynamic_Model_Fan_1_1_RIGID/LConn1
  Simulink-PS Converter/RConn1 -- External Force and Torque/LConn1
  DC Motor/RConn2 -- Im/RConn1
  Rev-Rot Interface1/LConn2 -- DC Motor/RConn1
  Revolute5/RConn2 -- Fan_p/RConn1
  Drag-Inertia Adj Prop Type/LConn1 -- Rev-Rot Interface1/RConn1 -- Revolute5/RConn3 -- PS Gain/LConn1
  Revolute5/LConn1 -- External Force and Torque/RConn1 -- x05_Aero_Dynamic_Model_Fan_1_Module_1_RIGID/RConn1
  x05_Aero_Dynamic_Model_Fan_1_Module_1_RIGID/LConn1 -- B/RConn1
  Rev-Rot Interface1/RConn2 -- Mechanical Rotational Reference2/LConn1
  PS Gain/RConn1 -- PS-Simulink Converter/LConn1 -- Fan_w/RConn1
  Drag-Inertia Adj Prop Type/RConn2 -- Rev-Rot Interface1/LConn1

== system Aero_Workspace/Virtual Aero/Simscape Multibody/Pivot ==
  angle_fan_y : Inport
  A002_759_1_RIGID : Subsystem
  C006_323_1_RIGID : Subsystem
  Pitch Fan Angle : sm_lib/Frames and Transforms/Rigid Transform  TranslationMethod=None  TranslationStandardOffset=0  TranslationLengthUnit=in  TranslationStandardAxis=+Z  TranslationCartesianOffset=smiData.RigidTransform(3).translation  TranslationROffset=0  TranslationROffsetUnits=m  TranslationZOffset=0  TranslationZOffsetUnits=m  TranslationThetaOffset=0  TranslationThetaOffsetUnits=deg  RotationMethod=StandardAxis  RotationAngleUnits=rad  RotationStandardAxis=-Z  RotationAngle=pi  RotationArbitraryAxis=smiData.RigidTransform(3).axis  FollAlignAxisA=+X  BaseAlignAxisA=+Y  FollAlignAxisB=+Y  BaseAlignAxisB=+Z  RotationSequenceAxes=FollowerAxes  RotationSequence=XZX  RotationSequenceAngles=[0 0 0]  RotationSequenceAnglesUnits=deg  RotationMatrix=[1 0 0; 0 1 0; 0 0 1]
  ReferenceFrame : sm_lib/Frames and Transforms/Reference Frame
  Revolute Joint : sm_lib/Joints/Revolute Joint  JointMode=Normal  SenseConstraintForce=off  SenseConstraintForceX=off  SenseConstraintForceY=off  SenseConstraintForceZ=off  SenseConstraintTorque=off  SenseConstraintTorqueX=off  SenseConstraintTorqueY=off  SenseConstraintTorqueZ=off  SenseTotalForce=off  SenseTotalForceX=off  SenseTotalForceY=off  SenseTotalForceZ=off  SenseTotalTorque=off  SenseTotalTorqueX=off  SenseTotalTorqueY=off  SenseTotalTorqueZ=off  CompositeWrenchDir=FollowerOnBase  CompositeWrenchFrame=BaseFrame  EquilibriumPosition=0  EquilibriumPositionUnits=deg  SpringStiffness=0  SpringStiffnessUnits=N*m/deg  DampingCoefficient=0  DampingCoefficientUnits=N*m/(deg/s)  TorqueActuationMode=ComputedTorque  MotionActuationMode=InputMotion  SensePosition=off  SenseVelocity=off  SenseAcceleration=off  SenseTorqueForce=off  SenseLowerLimitTorqueForce=off  SenseUpperLimitTorqueForce=off  LowerLimitSpecify=off  LowerLimitBound=-90  LowerLimitBoundUnits=deg  LowerLimitStiffness=1e4  LowerLimitStiffnessUnits=N*m/deg  LowerLimitDamping=10  LowerLimitDampingUnits=N*m/(deg/s)  LowerLimitTransitionRegionWidth=0.1  LowerLimitTransitionRegionWidthUnits=deg  UpperLimitSpecify=off  UpperLimitBound=90  UpperLimitBoundUnits=deg  UpperLimitStiffness=1e4  UpperLimitStiffnessUnits=N*m/deg  UpperLimitDamping=10  UpperLimitDampingUnits=N*m/(deg/s)  UpperLimitTransitionRegionWidth=0.1  UpperLimitTransitionRegionWidthUnits=deg  PositionTargetSpecify=off  PositionTargetPriority=High  PositionTargetValue=0  PositionTargetValueUnits=deg  VelocityTargetSpecify=off  VelocityTargetPriority=High  VelocityTargetValue=0  VelocityTargetValueUnits=deg/s
  Simulink-PS Converter : nesl_utility/Simulink-PS Converter  PhysicalDomain=network_engine_domain  SubClassName=ps_input  LeftPortType=input  RightPortType=output  PseudoPeriodic=off  Frequencies=[]  NoiseDistribution=none  NoiseParameters=[]  Unit=1  AffineConversion=off  FilteringAndDerivatives=zero  SimscapeFilterOrder=1  InputFilterTimeConstant=0.001  UdotUserProvided=1
      settings: SourceProductBaseCode=PW,SS
  Transform : sm_lib/Frames and Transforms/Rigid Transform  TranslationMethod=Cartesian  TranslationStandardOffset=0  TranslationLengthUnit=in  TranslationStandardAxis=+Z  TranslationCartesianOffset=smiData.RigidTransform(3).translation  TranslationROffset=0  TranslationROffsetUnits=m  TranslationZOffset=0  TranslationZOffsetUnits=m  TranslationThetaOffset=0  TranslationThetaOffsetUnits=deg  RotationMethod=ArbitraryAxis  RotationAngleUnits=rad  RotationStandardAxis=+Z  RotationAngle=smiData.RigidTransform(3).angle  RotationArbitraryAxis=smiData.RigidTransform(3).axis  FollAlignAxisA=+X  BaseAlignAxisA=+Y  FollAlignAxisB=+Y  BaseAlignAxisB=+Z  RotationSequenceAxes=FollowerAxes  RotationSequence=XZX  RotationSequenceAngles=[0 0 0]  RotationSequenceAnglesUnits=deg  RotationMatrix=[1 0 0; 0 1 0; 0 0 1]
  Transform1 : sm_lib/Frames and Transforms/Rigid Transform  TranslationMethod=Cartesian  TranslationStandardOffset=0  TranslationLengthUnit=in  TranslationStandardAxis=+Z  TranslationCartesianOffset=smiData.RigidTransform(6).translation  TranslationROffset=0  TranslationROffsetUnits=m  TranslationZOffset=0  TranslationZOffsetUnits=m  TranslationThetaOffset=0  TranslationThetaOffsetUnits=deg  RotationMethod=ArbitraryAxis  RotationAngleUnits=rad  RotationStandardAxis=+Z  RotationAngle=smiData.RigidTransform(6).angle  RotationArbitraryAxis=smiData.RigidTransform(6).axis  FollAlignAxisA=+X  BaseAlignAxisA=+Y  FollAlignAxisB=+Y  BaseAlignAxisB=+Z  RotationSequenceAxes=FollowerAxes  RotationSequence=XYX  RotationSequenceAngles=[0 0 0]  RotationSequenceAnglesUnits=deg  RotationMatrix=[1 0 0; 0 1 0; 0 0 1]
  Transform2 : sm_lib/Frames and Transforms/Rigid Transform  TranslationMethod=Cartesian  TranslationStandardOffset=0  TranslationLengthUnit=in  TranslationStandardAxis=+Z  TranslationCartesianOffset=smiData.RigidTransform(9).translation  TranslationROffset=0  TranslationROffsetUnits=m  TranslationZOffset=0  TranslationZOffsetUnits=m  TranslationThetaOffset=0  TranslationThetaOffsetUnits=deg  RotationMethod=ArbitraryAxis  RotationAngleUnits=rad  RotationStandardAxis=+Z  RotationAngle=smiData.RigidTransform(9).angle  RotationArbitraryAxis=smiData.RigidTransform(9).axis  FollAlignAxisA=+X  BaseAlignAxisA=+Y  FollAlignAxisB=+Y  BaseAlignAxisB=+Z  RotationSequenceAxes=FollowerAxes  RotationSequence=XYX  RotationSequenceAngles=[0 0 0]  RotationSequenceAnglesUnits=deg  RotationMatrix=[1 0 0; 0 1 0; 0 0 1]
  Transform3 : sm_lib/Frames and Transforms/Rigid Transform  TranslationMethod=Cartesian  TranslationStandardOffset=0  TranslationLengthUnit=in  TranslationStandardAxis=+Z  TranslationCartesianOffset=smiData.RigidTransform(417).translation  TranslationROffset=0  TranslationROffsetUnits=m  TranslationZOffset=0  TranslationZOffsetUnits=m  TranslationThetaOffset=0  TranslationThetaOffsetUnits=deg  RotationMethod=ArbitraryAxis  RotationAngleUnits=rad  RotationStandardAxis=+Z  RotationAngle=smiData.RigidTransform(417).angle  RotationArbitraryAxis=smiData.RigidTransform(417).axis  FollAlignAxisA=+X  BaseAlignAxisA=+Y  FollAlignAxisB=+Y  BaseAlignAxisB=+Z  RotationSequenceAxes=FollowerAxes  RotationSequence=XYX  RotationSequenceAngles=[0 0 0]  RotationSequenceAnglesUnits=deg  RotationMatrix=[1 0 0; 0 1 0; 0 0 1]
  B : PMIOPort  Side=Left
  F1 : PMIOPort  Port=2  Side=Right
  F0 : PMIOPort  Port=3  Side=Right
  wires:
  angle_fan_y/1 -> Simulink-PS Converter/1
  connections:
  Pitch Fan Angle/RConn1 -- F1/RConn1
  A002_759_1_RIGID/RConn1 -- ReferenceFrame/RConn1 -- Transform/LConn1 -- Transform1/LConn1 -- Transform2/LConn1 -- Transform3/LConn1
  Transform1/RConn1 -- B/RConn1
  Transform2/RConn1 -- Pitch Fan Angle/LConn1
  C006_323_1_RIGID/LConn1 -- Transform3/RConn1
  Transform/RConn1 -- Revolute Joint/LConn1
  Revolute Joint/RConn1 -- F0/RConn1
  Simulink-PS Converter/RConn1 -- Revolute Joint/LConn2

== system Aero_Workspace/Virtual Aero/Simscape Multibody/Yoke ==
  pitch_lock : Inport
  Mechanical Rotational Reference : fl_lib/Mechanical/Rotational Elements/Mechanical Rotational Reference
  Pitch Axis : sm_lib/Joints/Revolute Joint  JointMode=Normal  SenseConstraintForce=off  SenseConstraintForceX=off  SenseConstraintForceY=off  SenseConstraintForceZ=off  SenseConstraintTorque=off  SenseConstraintTorqueX=off  SenseConstraintTorqueY=off  SenseConstraintTorqueZ=off  SenseTotalForce=off  SenseTotalForceX=off  SenseTotalForceY=off  SenseTotalForceZ=off  SenseTotalTorque=off  SenseTotalTorqueX=off  SenseTotalTorqueY=off  SenseTotalTorqueZ=off  CompositeWrenchDir=FollowerOnBase  CompositeWrenchFrame=BaseFrame  EquilibriumPosition=0  EquilibriumPositionUnits=rad  SpringStiffness=Ksp  SpringStiffnessUnits=m*N/rad  DampingCoefficient=Dp  DampingCoefficientUnits=m*s*N/rad  TorqueActuationMode=InputTorque  MotionActuationMode=ComputedMotion  SensePosition=on  SenseVelocity=on  SenseAcceleration=off  SenseTorqueForce=off  SenseLowerLimitTorqueForce=off  SenseUpperLimitTorqueForce=off  LowerLimitSpecify=off  LowerLimitBound=-90  LowerLimitBoundUnits=deg  LowerLimitStiffness=1e4  LowerLimitStiffnessUnits=N*m/deg  LowerLimitDamping=10  LowerLimitDampingUnits=N*m/(deg/s)  LowerLimitTransitionRegionWidth=0.1  LowerLimitTransitionRegionWidthUnits=deg  UpperLimitSpecify=off  UpperLimitBound=90  UpperLimitBoundUnits=deg  UpperLimitStiffness=1e4  UpperLimitStiffnessUnits=N*m/deg  UpperLimitDamping=10  UpperLimitDampingUnits=N*m/(deg/s)  UpperLimitTransitionRegionWidth=0.1  UpperLimitTransitionRegionWidthUnits=deg  PositionTargetSpecify=off  PositionTargetPriority=Low  PositionTargetValue=smiData.RevoluteJoint(3).Rz.Pos  PositionTargetValueUnits=deg  VelocityTargetSpecify=off  VelocityTargetPriority=High  VelocityTargetValue=0  VelocityTargetValueUnits=deg/s
  Rev-Rot Interface : Subsystem
  Rotational Hard Stop : fl_lib/Mechanical/Rotational Elements/Rotational Hard Stop  upper_bnd=Pitch_deg_range deg  lower_bnd=-Pitch_deg_range deg  stiff_up=1e6 N*m/rad  stiff_low=1e6 N*m/rad  D_up=0.01 N*m/(rad/s)  D_low=0.01 N*m/(rad/s)  model=3  transition=0.001 rad  w_specify=off  w_priority=None  w=0 rad/s  w_nominal_specify=off  w_nominal_unit=rad/s  w_nominal_value=1  t_specify=off  t_priority=None  t=0 N*m  t_nominal_specify=off  t_nominal_unit=N*m  t_nominal_value=1  phi_specify=off  phi_priority=High  phi=0 rad  phi_nominal_specify=off  phi_nominal_unit=rad  phi_nominal_value=1
      settings: SourceProductBaseCode=SS
  x02_Aero_Dynamic_Model_Yoke_1_RIGID : Subsystem
  B : PMIOPort  Side=Left
  F : PMIOPort  Port=2  Side=Right
  Pitch_p : PMIOPort  Port=3  Side=Right
  Pitch_w : PMIOPort  Port=4  Side=Right
  wires:
  pitch_lock/1 -> Rev-Rot Interface/1(pitch_lock)
  connections:
  Rev-Rot Interface/LConn1 -- Pitch Axis/LConn2
  Rotational Hard Stop/RConn1 -- Mechanical Rotational Reference/LConn1 -- Rev-Rot Interface/RConn2
  Rev-Rot Interface/LConn2 -- Rotational Hard Stop/LConn1
  Pitch Axis/LConn1 -- x02_Aero_Dynamic_Model_Yoke_1_RIGID/RConn1
  Pitch Axis/RConn1 -- F/RConn1
  B/RConn1 -- x02_Aero_Dynamic_Model_Yoke_1_RIGID/LConn1
  Pitch Axis/RConn2 -- Pitch_p/RConn1
  Pitch Axis/RConn3 -- Rev-Rot Interface/RConn1 -- Pitch_w/RConn1

== system Aero_Workspace/Virtual Aero/Simscape Multibody/Back Rotor - Motor 1/DC Motor ==
  V : Inport
  Controlled Voltage Source : fl_lib/Electrical/Electrical Sources/Controlled Voltage Source
  Current Sensor : fl_lib/Electrical/Electrical Sensors/Current Sensor
  DC Motor : ee_lib/Electromechanical/Brushed Motors/DC Motor  field_option=ee.enum.field_option.pm  Rf=100 Ohm  Lf=1 H  Laf=0.15 H  If0=0 A  parameterization=ee.enum.dcparam_option.circuit_param  Ra=9.7564 Ohm  La=1.16 mH  emf_or_torque=ee.enum.emf_or_torque.kv  Kv=0.041 V/(rad/s)  Ki=6.876e-4 N*m/A  T_stall=0.24e-3 N*m  w_max=19100 rpm  w_rated=15000 rpm  P_rated=0.08 W  V_rated=1.5 V  J=4e-6 kg*m^2  lam_param=ee.enum.lam_param.damping  lam=2.6032e-7 N*m/(rad/s)  i_noload=0.022 A  V_i_noload=18 V  speed0=0 rpm  enable_fault_armature=ee.enum.faults.faultEnable.no  rev_faulted=1 / 3  G_faulted_armature=1e-5 S  fault_trigger_armature=ee.enum.faults.faultTrigger.temporal  t_fault_armature=1 s  max_permissible_current_armature=inf A  t_fail_on_current_armature=1 s  enable_fault_field=ee.enum.faults.faultEnable.no  G_faulted_field=1e-5 S  fault_trigger_field=ee.enum.faults.faultTrigger.temporal  t_fault_field=1 s  max_permissible_current_field=inf A  t_fail_on_current_field=1 s  fault_action=ee.enum.faults.faultAction.none  alpha=3.93e-3 1/K  Tmeas=25 degC  thermal_mass=100 J/K  initial_temperature=25 degC
  Electrical Reference : fl_lib/Electrical/Electrical Elements/Electrical Reference
  Friction : fl_lib/Mechanical/Rotational Elements/Rotational Friction  brkwy_trq=3e-4 N*m  brkwy_vel=1.6522e-06 rad/s  Col_trq=3e-4 N*m  visc_coef=2.6032e-7 N*m/(rad/s)  w_specify=off  w_priority=High  w=0 rad/s  w_nominal_specify=off  w_nominal_unit=rad/s  w_nominal_value=1  t_specify=off  t_priority=High  t=0 N*m  t_nominal_specify=off  t_nominal_unit=N*m  t_nominal_value=1
  Mechanical Rotational Reference : fl_lib/Mechanical/Rotational Elements/Mechanical Rotational Reference
  Simulink-PS Converter : nesl_utility/Simulink-PS Converter  PhysicalDomain=network_engine_domain  SubClassName=ps_input  LeftPortType=input  RightPortType=output  PseudoPeriodic=off  Frequencies=[]  NoiseDistribution=none  NoiseParameters=[]  Unit=1  AffineConversion=off  FilteringAndDerivatives=provide  SimscapeFilterOrder=1  InputFilterTimeConstant=0.001  UdotUserProvided=0
      settings: SourceProductBaseCode=PW,SS
  R : PMIOPort  Side=Right
  Im : PMIOPort  Port=2  Side=Right
  wires:
  V/1 -> Simulink-PS Converter/1
  connections:
  Friction/LConn1 -- R/RConn1 -- DC Motor/LConn2
  Friction/RConn1 -- DC Motor/RConn2 -- Mechanical Rotational Reference/LConn1
  DC Motor/RConn1 -- Controlled Voltage Source/RConn2 -- Electrical Reference/LConn1
  Simulink-PS Converter/RConn1 -- Controlled Voltage Source/RConn1
  Controlled Voltage Source/LConn1 -- Current Sensor/LConn1
  Current Sensor/RConn1 -- Im/RConn1
  Current Sensor/RConn2 -- DC Motor/LConn1
